simulink model "simulink_model"  (R2014b)
settings: Solver=ode45  StartTime=0.0  RelTol=1e-3
values from neighbouring files (symbols this model uses):
  X0 = [0 0 0   ]'    [main.m]
  Xdot0 = [0 0 0  ]'    [main.m]
undefined symbols (not defined in the file or in its folder): sigbuilder_block
settings Model: CovSFcnEnable=on  Creator=Jaby  LastModifiedBy=Raman
settings OptimizationCC: UseDivisionForNetSlopeComputation=off  SimCompilerOptimization=off
settings DebuggingCC: SolverPrmCheckMsg=none  FrameProcessingCompatibilityMsg=error
settings RTWCC: RTWCompilerOptimization=off

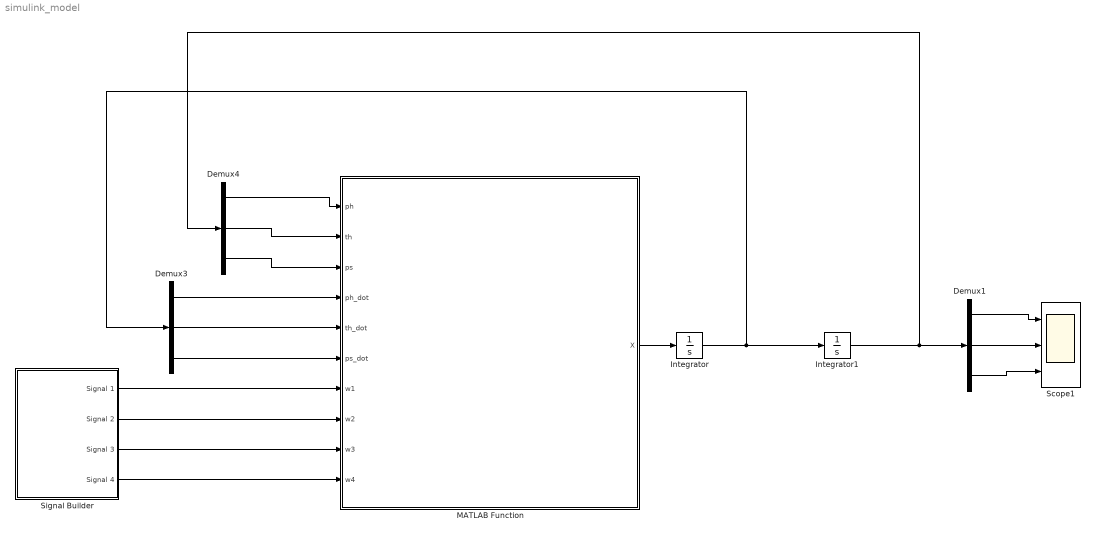
== system simulink_model ==
  Demux1 : Demux  Outputs=3
  Demux3 : Demux  Outputs=3
  Demux4 : Demux  Outputs=3
  Integrator : Integrator  InitialCondition=Xdot0
  Integrator1 : Integrator  InitialCondition=X0
  MATLAB Function : MATLAB Function  TreatAsAtomicUnit=on
  Scope1 : Scope  NumInputPorts=3
      settings: TimeRange=6  YMin=0~-5~-5  YMax=0.004~5~5
  Signal Builder : Subsystem  Tag=STV Subsys  LoadFcn=sigbuilder_block('load');  StartFcn=sigbuilder_block('start');  StopFcn=sigbuilder_block('stop');  ClipboardFcn=sigbuilder_block('clipboard');  mask(Sigbuilder block){}
      mask help: Simulink:masks:SigbuilderBlock_MD
      mask init:
      | if ~strcmp(get_param(bdroot(gcbh),'SimulationStatus'),'stopped') tuvar = sigbuilder_block('maskInit'); end
      settings: CopyFcn=sigbuilder_block('copy');  DeleteFcn=sigbuilder_block('delete');  ModelCloseFcn=sigbuilder_block('modelClose');  PreSaveFcn=sigbuilder_block('preSave');  PauseFcn=sigbuilder_block('pause');  ContinueFcn=sigbuilder_block('continue');  NameChangeFcn=sigbuilder_block('namechange');  OpenFcn=sigbuilder_block('open',[437.6 199.2 550.4 400 ]);  CloseFcn=sigbuilder_block('close');
      mask Display: plot(0, 0, 100, 100,[2, 2, 32, 32, 2], [68, 8, 8, 68, 68],[32, 2], [38, 38], [32, 19, 2],[53, 60, 44], [32, 17, 17, 2],[16, 16, 31, 31]);txt = getActiveGroup(gcbh);text(2, 100, txt,'verticalAlignment', 'top');
  wires:
  MATLAB Function/1(X) -> Integrator/1
  Integrator/1 -> Demux3/1, Integrator1/1
  Integrator1/1 -> Demux1/1, Demux4/1
  Demux4/1 -> MATLAB Function/1(ph)
  Demux4/2 -> MATLAB Function/2(th)
  Demux4/3 -> MATLAB Function/3(ps)
  Demux3/1 -> MATLAB Function/4(ph_dot)
  Demux3/2 -> MATLAB Function/5(th_dot)
  Demux3/3 -> MATLAB Function/6(ps_dot)
  Demux1/2 -> Scope1/2
  Demux1/1 -> Scope1/1
  Demux1/3 -> Scope1/3
  Signal Builder/2(Signal 2) -> MATLAB Function/8(w2)
  Signal Builder/1(Signal 1) -> MATLAB Function/7(w1)
  Signal Builder/3(Signal 3) -> MATLAB Function/9(w3)
  Signal Builder/4(Signal 4) -> MATLAB Function/10(w4)

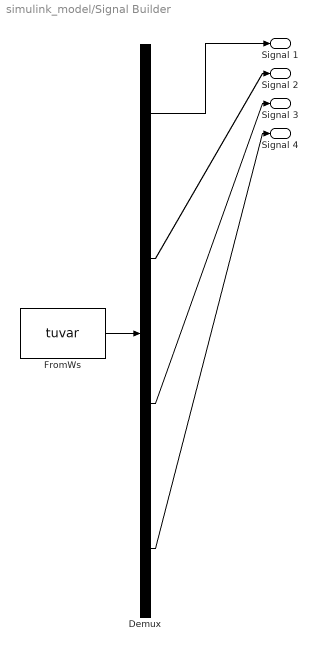
== system simulink_model/Signal Builder ==
  Demux : Demux  Tag=STV Demux
  FromWs : FromWorkspace  Tag=STV FromWs  VariableName=tuvar  SampleTime=0
      SigBuilderData=|
      | common.afterFinalStr = 'Extrapolate'
      | common.sampleTime = 0
      | dataSet.timeRange = [0 10]
      | dataSet.name = 'Group 1'
      | sbobj.Groups.Name = 'Group 1'
      | sbobj.Groups.Signals(1).Name = 'Signal 1'
      | sbobj.Groups.Signals(1).XData = [0 7.82 9.28 10]
      | sbobj.Groups.Signals(1).YData = [0 0 0 0]
      | sbobj.Groups.Signals(2).Name = 'Signal 2'
      | sbobj.Groups.Signals(2).XData = [0 2 2 2.1 2.1 10]
      | sbobj.Groups.Signals(2).YData = [0 0 1 1 0 0]
      | sbobj.Groups.Signals(3).Name = 'Signal 3'
      | sbobj.Groups.Signals(3).XData = [0 5.8 6 10]
      | sbobj.Groups.Signals(3).YData = [0 0 0 0]
      | sbobj.Groups.Signals(4).Name = 'Signal 4'
      | sbobj.Groups.Signals(4).XData = [0 2 2 2.1 2.1 10]
      | sbobj.Groups.Signals(4).YData = [0 0 1 1 0 0]
  Signal 1 : Outport  Tag=STV Outport
  Signal 2 : Outport  Tag=STV Outport  Port=2
  Signal 3 : Outport  Tag=STV Outport  Port=3
  Signal 4 : Outport  Tag=STV Outport  Port=4
  wires:
  Demux/1 -> Signal 1/1
  FromWs/1 -> Demux/1
  Demux/2 -> Signal 2/1
  Demux/3 -> Signal 3/1
  Demux/4 -> Signal 4/1

== matlab function simulink_model/MATLAB Function ==
  data: ph input; X output; th input; ps input; ph_dot input; th_dot input; ps_dot input; w1 input; w2 input; w3 input; w4 input
function  X= model(ph, th, ps, ph_dot,th_dot,ps_dot, w1,w2,w3,w4)

% Angular momentum
ixx = 0.14e-6;
iyy = 0.14e-6;
izz = 0.217e-6;

% Constants
L = 0.046; % Length
k = 2.75e-11; % Lift const
b = 1e-9; % Drag const
m = 26e-3; % Mass
ir = 1;
g = 9.81; % Gravity

% The angles
% ph = q(1);
% th =q(2);
% ps =q(3);

% Angular velocity
% ph_dot = qdot(1);
% th_dot = qdot(2);
% ps_dot = qdot(3);

% w1 = f(1);
% w2 = u(2);
% w3 = u(3);
% w4 = u(4);

% The torques
WT = w1 - w2 + w3 - w4;
T_th = L * k * (w2^2 + w3^2 - w1^2 - w4^2);
T_ph = L* k * (w3^2 + w4^2- w1^2 - w2^2);
T_ps = b * (w1^2 - w2^2 + w3^2 - w4^2);
T = k * (w1^2 + w2^2 + w3^2 + w4^2);

% Rotation matrix (body frame -> inertial frame)
R_TB = (T / m) * [cos(ps) * sin(th) * cos(ph) + sin(ps) * sin(ph);...
                  sin(ps) * sin(th) * cos(ph) - cos(ps) * sin(ph);...
                  cos(th) * cos(ph)];

% Linear acceleration
% x_ddot = R_TB(1);
% y_ddot = R_TB(2);
% z_ddot = -g + R_TB(3);
% state_tr = [x_ddot; y_ddot; z_ddot];

% Transormation matrix (body frame -> inertial frame)
wn_inv = [1, sin(ph) * tan(th), cos(ph) * tan(th);...
          0, cos(ph), -sin(ph);...
          0, sin(ph) / cos(th), cos(ph) / cos(th)];

% Angular velocity (inertial frame)
eta_dot = [ph_dot; th_dot; ps_dot];

% Angular velocity (body frame)
v =  [1, 0, -sin(th);...
      0, cos(ph), cos(th) * sin(ph);...
      0, -sin(ph), cos(th) * cos(ph)] * eta_dot;

p = v(1);
q = v(2);
r = v(3);


% Angular acceleration (body frame)
v_dot = [(iyy - izz) * q * r / ixx;...
         (izz - ixx) * p * r / iyy;...
         (ixx - iyy) * p * q / izz]...
         -ir * [q / ixx; -p / iyy; 0] * WT + [T_ph / ixx; T_th / iyy; T_ps / izz];

% v = [p; q; r];
% Angular acceleration (inertial frame)
eta_ddot = [0, ph_dot * cos(ph) * tan(th) + th_dot * sin(ph) / cos(th)^2,...
                -ph_dot * sin(ph) * cos(th) + th_dot * cos(ph) / cos(th)^2;...
            0, -ph_dot * sin(ph), -ph_dot * cos(ph);...
            0, ph_dot * cos(ph) / cos(th) + ph_dot * sin(ph) * tan(th) / cos(th),...
                -ph_dot * sin(ph) / cos(th) + th_dot * cos(ph) * tan(th) / cos(th)] * v+  wn_inv*v_dot;

% Function output
X=eta_ddot;
end
